simulink model "SwitchCaseLianxi"  (Simulink 9.1)
settings: Solver=VariableStepAuto  StartTime=0.0  StopTime=5  RelTol=1e-3
libraries: simulink x1
settings Model: Creator=McQueen_Zero  LastModifiedBy=McQueen_Zero
settings DataIOCC: SaveFormat=Dataset
settings OptimizationCC: LifeSpan=auto
settings DebuggingCC: UnderspecifiedInitializationDetection=Simplified  MergeDetectMultiDrivingBlocksExec=error  SFUnexpectedBacktrackingDiag=error  SFNoUnconditionalDefaultTransitionDiag=error  SFExecutionAtInitializationDiag=warning
settings HardwareCC: ProdBitPerPointer=64  ProdBitPerSizeT=64  ProdBitPerPtrDiffT=64  ProdLargestAtomicFloat=Float  ProdIntDivRoundTo=Zero  ProdEndianess=LittleEndian  ProdWordSize=64  ProdHWDeviceType=Intel->x86-64 (Windows64)
settings ModelReferenceCC: PropagateSignalLabelsOutOfModel=on
settings CodeAppCC: StateflowObjectComments=off
settings GRTTargetCC: TargetLangStandard=C99 (ISO)  CombineOutputUpdateFcns=on  GRTInterface=off
settings ConfigComp: CovMetricSettings=dwe  CovHtmlReporting=off  CovSaveCumulativeToWorkspaceVar=off  CovSaveSingleToWorkspaceVar=off  CovExternalEMLEnable=on

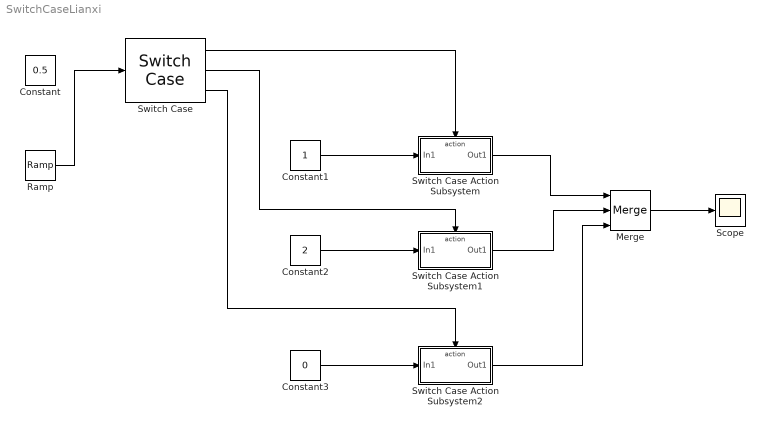
== system SwitchCaseLianxi ==
  Constant : Constant  Value=0.5
  Constant1 : Constant
  Constant2 : Constant  Value=2
  Constant3 : Constant  Value=0
  Merge : Merge  Inputs=3
  Ramp : simulink/Sources/Ramp  slope=1  start=0  InitialOutput=0
  Scope : Scope
  Switch Case : SwitchCase  CaseConditions={1,[2,3]}
  Switch Case Action Subsystem : Subsystem  TreatAsAtomicUnit=on
  Switch Case Action Subsystem1 : Subsystem  TreatAsAtomicUnit=on
  Switch Case Action Subsystem2 : Subsystem  TreatAsAtomicUnit=on
  wires:
  Merge/1 -> Scope/1
  Switch Case Action Subsystem/1(Out1) -> Merge/1
  Switch Case Action Subsystem1/1(Out1) -> Merge/2
  Switch Case Action Subsystem2/1(Out1) -> Merge/3
  Constant1/1 -> Switch Case Action Subsystem/1(In1)
  Constant2/1 -> Switch Case Action Subsystem1/1(In1)
  Constant3/1 -> Switch Case Action Subsystem2/1(In1)
  Ramp/1 -> Switch Case/1
  Switch Case/1 -> Switch Case Action Subsystem/Action
  Switch Case/2 -> Switch Case Action Subsystem1/Action
  Switch Case/3 -> Switch Case Action Subsystem2/Action

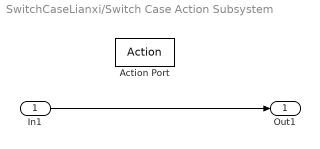
== system SwitchCaseLianxi/Switch Case Action Subsystem ==
  In1 : Inport
  Action Port : ActionPort  ActionType=case
  Out1 : Outport
  wires:
  In1/1 -> Out1/1

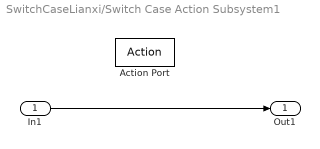
== system SwitchCaseLianxi/Switch Case Action Subsystem1 ==
  In1 : Inport
  Action Port : ActionPort  ActionType=case
  Out1 : Outport
  wires:
  In1/1 -> Out1/1

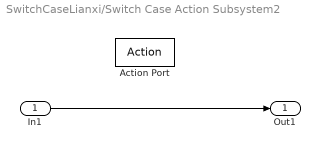
== system SwitchCaseLianxi/Switch Case Action Subsystem2 ==
  In1 : Inport
  Action Port : ActionPort  ActionType=default
  Out1 : Outport
  wires:
  In1/1 -> Out1/1
